simulink model "v2021_10_27_Modello_SITL_AENEA_2020b"  (R2022a)
settings: Solver=ode4  StartTime=0.0  StopTime=10  FixedStep=0.01  RelTol=1e-3
values from neighbouring files (symbols this model uses):
  alphavec_rad = deg2rad(alphavec)    [v2021_10_27_calcoloAerodinamica.m]
  attuatore_Amax = 20*(pi/180)    (= 0.349065850399)    [v2021_10_27_avvioSITL.m]    (also in v2021_10_27_calcoloAerodinamica.m)
  attuatore_Emax = 25*(pi/180)    (= 0.436332312999)    [v2021_10_27_avvioSITL.m]    (also in v2021_10_27_calcoloAerodinamica.m)
  attuatore_Rmax = 25*(pi/180)    (= 0.436332312999)    [v2021_10_27_avvioSITL.m]    (also in v2021_10_27_calcoloAerodinamica.m)
  b = 2.62    [AENEA2.m]    (also in v2021_10_27_calcoloAerodinamica.m)
  betavec_rad = deg2rad(betavec)    [v2021_10_27_calcoloAerodinamica.m]
  c = .32    (= 0.32)    [AENEA2.m]    (also in calcoloPolari.m = dim(2); v2021_10_27_calcoloAerodinamica.m)
  cbar = .32    (= 0.32)    [v2021_10_27_calcoloAerodinamica.m]
  CD0 = 0.024    [v2021_10_27_calcoloAerodinamica.m]
  CldA = KCldA(1)*180/pi    [AENEA2.m]
  CLdE = KCLdE(1)*180/pi    [AENEA2.m]
  CldR = KCldR(1)*180/pi    [AENEA2.m]
  Clp = -0.4318    [v2021_10_27_calcoloAerodinamica.m]
  CLq = 8.13    [v2021_10_27_calcoloAerodinamica.m]
  Clr = 0.1459    [v2021_10_27_calcoloAerodinamica.m]
  CmdE = KCmdE(1)*180/pi    [AENEA2.m]
  Cmq = -23.24    [v2021_10_27_calcoloAerodinamica.m]
  CndA = KCndA(1)*180/pi    [AENEA2.m]
  CndR = KCndR(1)*180/pi    [AENEA2.m]
  Cnp = 0.007507    [v2021_10_27_calcoloAerodinamica.m]
  Cnr = -0.4872    [v2021_10_27_calcoloAerodinamica.m]
  CYp = 0.050728    [v2021_10_27_calcoloAerodinamica.m]
  CYr = 0.358925    [v2021_10_27_calcoloAerodinamica.m]
  deltaAtrim = 0    [v2021_10_27_avvioSITL.m]
  deltaEtrim = 0    [v2021_10_27_avvioSITL.m]
  deltaRtrim = 0    [v2021_10_27_avvioSITL.m]
  deltaTtrim = 0.1    [v2021_10_27_avvioSITL.m]
  Dprop = 2*Rprop    (= 0.5334)    [v2021_10_27_calcoloAerodinamica.m]
  F = [                                     1, 0,            -(dt*vn)/(a + h)^2, dt/(a + h),                     0,   0,  0,  0,  0, 0, 0, 0, 0, 0, 0, 0, 0, 0 ... (first row only)    [jac_F_F1B.m]
  g = [0 0 9.81]'    [v2021_10_27_calcoloAerodinamica.m]
  HINI = -State0.Pos0(3)    [v2021_10_27_avvioSITL.m]
  Jeng = 0    [v2021_10_27_calcoloAerodinamica.m]
  Jprop = mprop*(Dprop^2)/12    (= 0.00422031414)    [v2021_10_27_calcoloAerodinamica.m]
  latitudineINI = 41.854432*pi/180    (= 0.730497644952)    [v2021_10_27_avvioSITL.m]
  longitudineINI = 12.306650*pi/180    (= 0.214791562391)    [v2021_10_27_avvioSITL.m]
  PWM_Aileron = rad2deg(deltaAtrim)*9+1503    [v2021_10_27_avvioSITL.m]
  PWM_Elevator = rad2deg(deltaEtrim)*(447/50)+(3007/2)    [v2021_10_27_avvioSITL.m]
  PWM_Rudder = rad2deg(deltaRtrim)*(447/50)+(3007/2)    [v2021_10_27_avvioSITL.m]
  PWM_Throttle = (deltaTtrim)*800+1100    (= 1180)    [v2021_10_27_avvioSITL.m]
  q = prediction(11)    [jac_F_F1B.m]
  r = dim(1)    [calcoloPolari.m]    (also in jac_F_F1B.m = prediction(12))
  rACtG = rACtP-rGP    [v2021_10_27_calcoloAerodinamica.m]
  rACwG = rACwP-rGP    [v2021_10_27_calcoloAerodinamica.m]
  rAHRSG = rAHRSP-rGP    [v2021_10_27_calcoloAerodinamica.m]
  rho = P/(287.05*T)    (= 1.16123787958)    [AENEA2.m]    (also in modello_appr_long.m = 1.164; v2021_10_27_calcoloAerodinamica.m = 1.2133)
  rLEG = rLEP-rGP    [v2021_10_27_calcoloAerodinamica.m]
  rmglG = rmglP-rGP    [v2021_10_27_calcoloAerodinamica.m]
  rmgrG = rmgrP-rGP    [v2021_10_27_calcoloAerodinamica.m]
  rngG = rngP-rGP    [v2021_10_27_calcoloAerodinamica.m]
  rNPG = rNPP-rGP    [v2021_10_27_calcoloAerodinamica.m]
  rPG = -rGP    [v2021_10_27_calcoloAerodinamica.m]
  Rprop = 0.2667    [v2021_10_27_calcoloAerodinamica.m]
  S = b*c    (= 0.8384)    [AENEA2.m]    (also in v2021_10_27_calcoloAerodinamica.m)
  sensori_FreqCampionamento_pitot = 0.02    [v2021_10_27_avvioSITL.m]
  sensori_RumoreSampleTime = 0.02    [v2021_10_27_avvioSITL.m]
  sensori_varianza = 0.0000    (= 0)    [v2021_10_27_avvioSITL.m]
  tsamp = 0.02    [v2021_10_27_avvioSITL.m]
  V_cruise = input('inserire un valore desiderato per V_cruise [m/s]: ')    [v2021_10_27_trimCalc.m]
  W = m*g    [v2021_10_27_calcoloAerodinamica.m]
  WP_AL = [     0 20 0 0 41.807822 12.589274 3 ... (first row only)    [v2021_10_27_avvioSITL.m]
  WP_db_info = [0 0 0 0 1 3;              0 0 0 0 2 3;              0 0 0 0 3 3;              0 0 0 0 0 0]    [v2021_10_27_avvioSITL.m]
  WP_db_param = [ ... (first row only)    [v2021_10_27_avvioSITL.m]
  Zeng = rPG(3)    [v2021_10_27_calcoloAerodinamica.m]
  Zpista = 0    [v2021_10_27_avvioSITL.m]
undefined symbols (not defined in the file or in its folder): beta_phi, beta_psi, beta_theta, CYdA, CYdR, delay_ahrs, delay_bmp, delay_gps, Earth, h_home, J_vec, matricepolinomi, mean_ax, mean_ay, mean_az, mean_p, mean_q, mean_r, MIL, P_ref, Receive, seed_ahrs, seed_baro, seed_gps, Send, State0, Std_con_lat, Std_con_long, Std_vel, T0_ref, Ta_lat, Ta_long, Ts_ahrs, Ts_bmp, Ts_gps, Var_heading_static, Var_V_hor_static, WGS84, White_ax, White_ay, White_az, White_gm_phi, White_gm_psi, White_gm_theta, White_p, White_pressione, White_r
libraries: simulink_extras x27, aerolibfltsims x5, aerolibwind2 x3, aerolibasang x2, simulink x2, shared6dof x1, slpidlib x1, aerolibatmos2 x1, aerolibanimutils x1
(part 1 of 3)
settings Model: Creator=Giorgio  LastModifiedBy=mvisc
settings SolverCC: AlgebraicLoopSolver=TrustRegion
settings DataIOCC: ReturnWorkspaceOutputs=off
settings DebuggingCC: ParameterPrecisionLossMsg=none  UnconnectedInputMsg=warning  UnconnectedOutputMsg=warning  UnconnectedLineMsg=warning  BusObjectLabelMismatch=none  SFMachineParentedDataDiag=warning  ArithmeticOperatorsInVariantConditions=warning
settings SFSimCC: CustomCodeUndefinedFunction=UseInterfaceOnly
settings RTWCC: DLArmComputeVersion=19.05

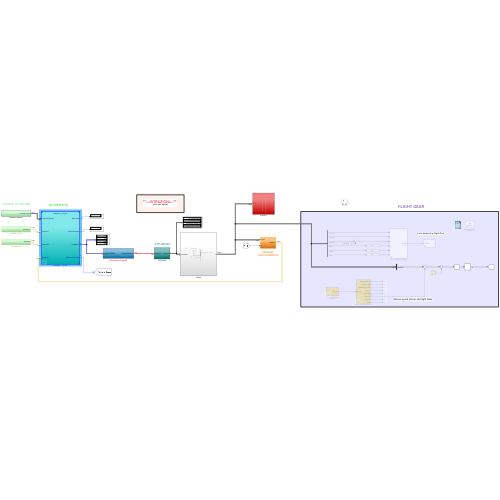
[thumbnail: Simulink's stored preview of the top-level diagram]
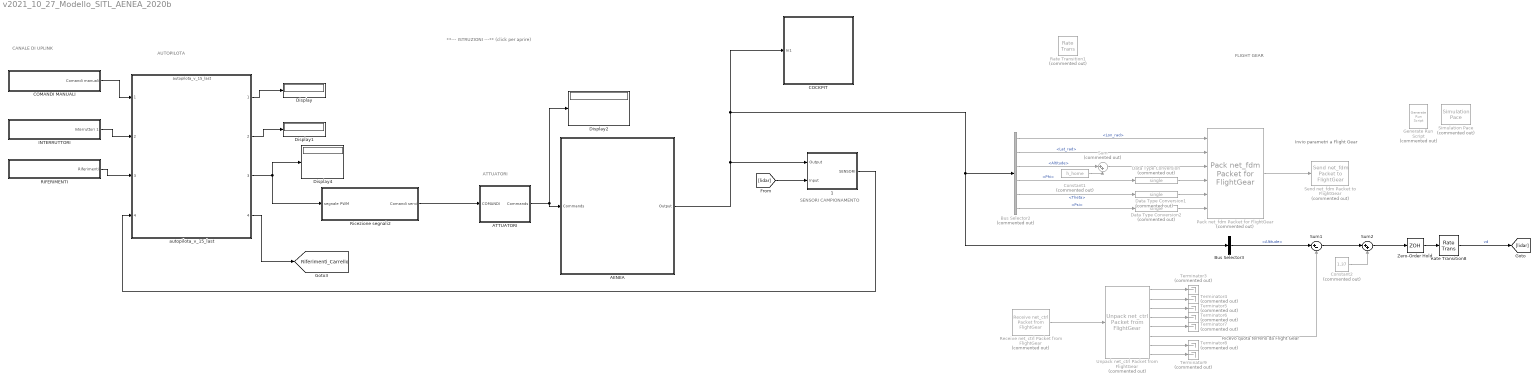
== system v2021_10_27_Modello_SITL_AENEA_2020b ==
  note: AUTOPILOTA
  note: SENSORI
      | CAMPIONAMENTO
  note: ATTUATORI
  note: CANALE DI UPLINK
  note: Ricevo quota terreno da Flight Gear
  note: Invio parametri a Flight Gear
  note: FLIGHT GEAR
  note: **--- ISTRUZIONI ---**
      | (click per aprire)
  " 1" : Subsystem
  "AENEA " : Subsystem
  ATTUATORI : Subsystem
  Bus Selector2 : BusSelector  Commented=on  OutputSignals=Lon_rad,Lat_rad,Altitude,Phi,Theta,Psi
  Bus Selector3 : BusSelector  OutputSignals=Altitude
  COCKPIT : Subsystem
  COMANDI MANUALI : Subsystem
  Constant1 : Constant  Commented=on  Value=h_home
  Constant2 : Constant  Commented=on  Value=1.37
  Data Type Conversion : DataTypeConversion  Commented=on  OutDataTypeStr=single  SaturateOnIntegerOverflow=off  RndMeth=Floor
  Data Type Conversion1 : DataTypeConversion  Commented=on  OutDataTypeStr=single  SaturateOnIntegerOverflow=off  RndMeth=Floor
  Data Type Conversion2 : DataTypeConversion  Commented=on  OutDataTypeStr=single  SaturateOnIntegerOverflow=off  RndMeth=Floor
  Display{,1..2,4} (4 alike) : Display
  Generate Run Script : aerolibfltsims/Generate Run Script  Commented=on  Architecture=Default  dataFlow=Send-Receive  GeometryModelName=c172p  AirportId=LIRF  RunwayId=34L  InitialAltitude=0  InitialHeading=340  OffsetDistance=0  OffsetAzimuth=0  InstallScenery=off  DisableShaders=off  OriginAddress=127.0.0.1  DestinationPort=5502  OriginPort=5505  LocalAddress=127.0.0.1  OutputFileName=runfg_sr.bat  FlightGearBaseDirectory=C:\Program Files\FlightGear 2016.1.2
  "INTERRUTTORI " : Subsystem
  Pack net_fdm Packet for FlightGear : aerolibfltsims/Pack net_fdm Packet for FlightGear  Commented=on  FlightGearVersion=v2016.1  ShowPositionAttitudeInputs=on  ShowVelocityAccelerationInputs=off  ShowControlSurfacePositionInputs=off  ShowEngineFuelInputs=off  ShowLandingGearInputs=off  ShowEnvironmentInputs=off  SampleTime=-1  packetVersion=24
      settings: SourceProductBaseCode=AE
  RIFERIMENTI : Subsystem
  Rate Transition1 : RateTransition  Commented=on  InitialCondition=[PWM_Throttle PWM_Elevator PWM_Aileron PWM_Rudder]
  Rate Transition8 : RateTransition  Deterministic=off  InitialCondition=State0.Pos0(3)  OutPortSampleTime=0.02
  Receive net_ctrl Packet from FlightGear : aerolibfltsims/Receive net_ctrl Packet from FlightGear  Commented=on  FlightGearVersion=v2016.1  ReceiveAddress=127.0.0.1  ReceivePort=5505  ReceiveWidth=744  varLen=off  SampleTime=-1  packetFlag=off
      settings: AttributesFormatString=Version Selected:\n%<FlightGearVersion>  SourceProductBaseCode=AE
  Ricezione segnali2 : Subsystem
  Send net_fdm Packet to FlightGear : aerolibfltsims/Send net_fdm Packet to FlightGear  Commented=on  DestinationIpAddress=127.0.0.1  DestinationPort=5502  LocalIpPort=-1  varLen=off  SampleTime=-1
      settings: SourceProductBaseCode=AE
  Simulation Pace : aerolibanimutils/Simulation Pace  Commented=on  SimulationPace=1  SleepMode=MATLAB Thread  OutputPaceError=off  SampleTime=tsamp
  Sum : Sum  Commented=on  Inputs=|++
  Sum1 : Sum  Inputs=|+-
  Sum2 : Sum  Inputs=|++
  Terminator{3..9} (7 alike) : Terminator  Commented=on
  Unpack net_ctrl Packet from FlightGear : aerolibfltsims/Unpack net_ctrl Packet from FlightGear  Commented=on  FlightGearVersion=v2016.1  ShowControlSurfacePositionOutputs=off  ShowEngineFuelOutputs=off  ShowLandingGearOutputs=off  ShowAvionicOutputs=off  ShowEnvironmentOutputs=on  SampleTime=-1  packetVersion=27
      settings: AttributesFormatString=Version Selected: %<FlightGearVersion>  SourceProductBaseCode=AE
  Zero-Order Hold : ZeroOrderHold  SampleTime=0.02
  autopilota_v_15_last : ModelReference  ModelNameDialog=autopilota_v_15_last.slx  SimulationMode=Normal  ModelReferenceVersion=8.0
  tag scope: Riferimenti_Carrello=global
  wires:
  autopilota_v_15_last/1 -> Display/1
  "INTERRUTTORI "/1(Interruttori 1) -> autopilota_v_15_last/2
  COMANDI MANUALI/1(Comandi manuali) -> autopilota_v_15_last/1
  autopilota_v_15_last/2 -> Display1/1
  RIFERIMENTI/1(Riferimenti) -> autopilota_v_15_last/3
  Constant2/1 -> Sum2/2
  Bus Selector2/6 -> Data Type Conversion2/1  "<Psi>"
  Bus Selector2/3 -> Sum/1  "<Altitude>"
  Sum1/1 -> Sum2/1
  Unpack net_ctrl Packet from FlightGear/6 -> Sum1/2
  Unpack net_ctrl Packet from FlightGear/2 -> Terminator4/1
  Unpack net_ctrl Packet from FlightGear/7 -> Terminator8/1
  Rate Transition8/1 -> [lidar]  "vd"
  Receive net_ctrl Packet from FlightGear/1 -> Unpack net_ctrl Packet from FlightGear/1
  Sum2/1 -> Zero-Order Hold/1
  Unpack net_ctrl Packet from FlightGear/8 -> Terminator9/1
  Bus Selector2/2 -> Pack net_fdm Packet for FlightGear/2  "<Lat_rad>"
  Constant1/1 -> Sum/2
  Data Type Conversion2/1 -> Pack net_fdm Packet for FlightGear/6
  Bus Selector3/1 -> Sum1/1  "<Altitude>"
  Unpack net_ctrl Packet from FlightGear/3 -> Terminator5/1
  Pack net_fdm Packet for FlightGear/1 -> Send net_fdm Packet to FlightGear/1
  Zero-Order Hold/1 -> Rate Transition8/1
  Data Type Conversion/1 -> Pack net_fdm Packet for FlightGear/4
  Sum/1 -> Pack net_fdm Packet for FlightGear/3
  Bus Selector2/4 -> Data Type Conversion/1  "<Phi>"
  Bus Selector2/5 -> Data Type Conversion1/1  "<Theta>"
  Unpack net_ctrl Packet from FlightGear/1 -> Terminator3/1
  Data Type Conversion1/1 -> Pack net_fdm Packet for FlightGear/5
  Bus Selector2/1 -> Pack net_fdm Packet for FlightGear/1  "<Lon_rad>"
  Unpack net_ctrl Packet from FlightGear/4 -> Terminator6/1
  Unpack net_ctrl Packet from FlightGear/5 -> Terminator7/1
  [lidar] -> " 1"/2(Input)
  "AENEA "/1(Output) -> " 1"/1(Output), Bus Selector3/1, Bus Selector2/1, COCKPIT/1(In1)
  ATTUATORI/1(Commands) -> "AENEA "/1(Commands), Display2/1
  autopilota_v_15_last/3 -> Display4/1, Ricezione segnali2/1(segnale PWM)
  Ricezione segnali2/1(Comandi servi) -> ATTUATORI/1("COMANDI ")
  " 1"/1(SENSORI) -> autopilota_v_15_last/4
  autopilota_v_15_last/4 -> [Riferimenti_Carrello]

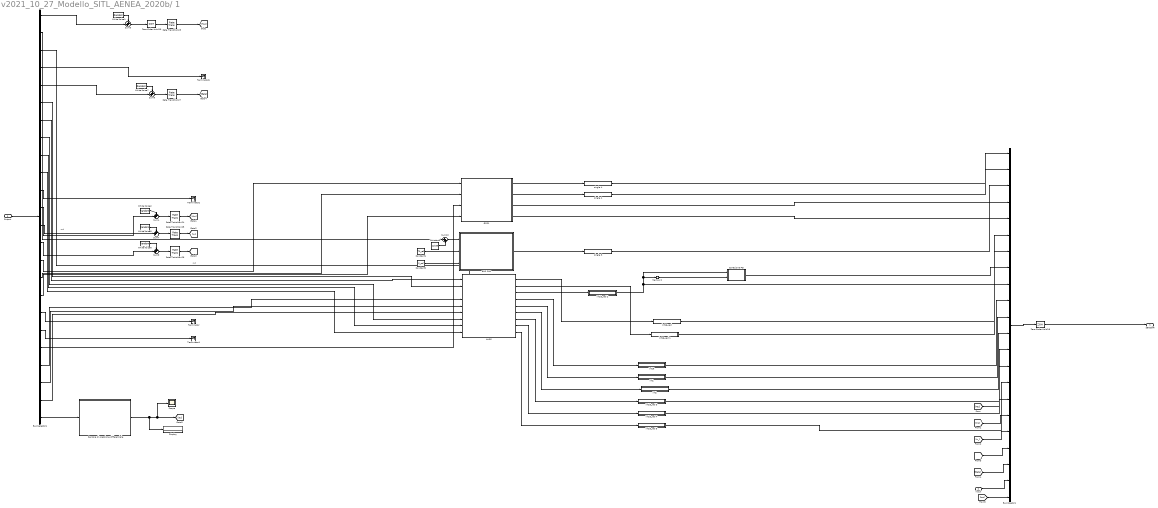
== system v2021_10_27_Modello_SITL_AENEA_2020b/ 1 ==
  note: rad
  note: rad
  Output : Inport
  Input : Inport  Port=2
  AHRS : Subsystem
  BMP 280 : Subsystem
  Bus Creator1 : BusCreator  Inputs=22  OutDataTypeStr=Bus: slBus8_sensori2
  Bus Selector1 : BusSelector  OutputSignals=V,Altitude,Psi,α,β,Theta,Phi,p,q,r,Zepunto,rho,w,Omega,Lat_rad,Lon_rad,heading,Xepunto,Yepunto,GS,upunto,vpunto,wpunto,deltaP
  Constant1 : Constant  Value=T0_ref
  Constant2 : Constant  Value=P_ref
  Constant3 : Constant  Value=Zpista
  Correzione PSI : MATLAB Function  TreatAsAtomicUnit=on
  Display : Display
  GPS1 : Subsystem
  Memory2 : Memory
  Rate Transition23 : RateTransition  OutPortSampleTime=0.02
  Rate Transition{24..27} (4 alike) : RateTransition  OutPortSampleTimeOpt=Inherit
  Scope : Scope
  Sensore di pressione differenziale : Subsystem
  Sum10 : Sum  Inputs=|++
  Sum{3..4,7..9} (5 alike) : Sum  Inputs=++|
  Terminator{,1..2,6} (4 alike) : Terminator
  White Noise1 : RandomNumber  DisableCoverage=on  Variance=1e-1  Seed=[23341]  SampleTime=sensori_RumoreSampleTime
  White Noise{2,5..7} (4 alike) : RandomNumber  DisableCoverage=on  Variance=sensori_varianza  Seed=[23341]  SampleTime=sensori_RumoreSampleTime
  Zero-Order Hold18 : ZeroOrderHold  SampleTime=0.02
  Zero-Order Hold19 : ZeroOrderHold  SampleTime=sensori_FreqCampionamento_pitot
  int1 : Subsystem
  int16 : Subsystem
  "int16_rad " : Subsystem
  int16_rad 1 : Subsystem
  int16_rad 2 : Subsystem
  int16_rad 3 : Subsystem
  int16_rad 4 : Subsystem
  int16_rad 5 : Subsystem
  int2 : Subsystem
  single 1 : Subsystem
  single 3 : Subsystem
  single 4 : Subsystem
  SENSORI : Outport  OutDataTypeStr=double  VectorParamsAs1DForOutWhenUnconnected=off
  wires:
  GPS1/3(V_n) -> Bus Creator1/4  "vn"
  Bus Selector1/19 -> Terminator1/1  "<Yepunto>"
  Bus Selector1/6 -> AHRS/2(theta)  "<Theta>"
  Bus Selector1/4 -> Terminator6/1  "<α>"
  Bus Selector1/23 -> AHRS/6(az)  "<wpunto>"
  Bus Selector1/18 -> Terminator/1  "<Xepunto>"
  Bus Selector1/2 -> Sum10/1  "<Altitude>"
  Bus Selector1/16 -> GPS1/2(Long)  "<Lon_rad>"
  Bus Selector1/17 -> GPS1/4(head)  "<heading>"
  Bus Selector1/7 -> AHRS/1(phi)  "<Phi>"
  Bus Selector1/22 -> AHRS/5(ay)  "<vpunto>"
  Bus Selector1/10 -> AHRS/9(r)  "<r>"
  GPS1/1(Lat_out) -> single 4/1(<u>)  "Lat"
  Rate Transition27/1 -> [Beta]  "Beta"
  "int16_rad "/1(Out1) -> Bus Creator1/6  "phi"
  Bus Selector1/5 -> Sum9/2  "<β>"
  White Noise2/1 -> Sum4/1
  White Noise5/1 -> Sum7/1
  AHRS/7(p_out) -> int16_rad 3/1(In1)  "p"
  Sum4/1 -> Rate Transition24/1  "rho"
  int16/1(Out1) -> Bus Creator1/10  "ax"
  Bus Selector1/14 -> Sum8/2  "<Omega>"
  BMP 280/1(quota_out) -> single 3/1(<u>)  "Alt"
  AHRS/4(ax_out) -> int16/1(In1)  "ax"
  Rate Transition25/1 -> [w_]  "w"
  int16_rad 5/1(Out1) -> Bus Creator1/15  "r"
  AHRS/6(az_out) -> int2/1(In1)  "az"
  GPS1/4(V_e) -> Bus Creator1/5  "ve"
  Bus Selector1/12 -> Sum4/2  "<rho>"
  Constant1/1 -> BMP 280/2(T0_ref)
  Bus Selector1/8 -> AHRS/7(p)  "<p>"
  Sum7/1 -> Rate Transition25/1  "w"
  Output/1 -> Bus Selector1/1
  Sum3/1 -> Zero-Order Hold19/1  "Tas"
  Bus Selector1/11 -> Terminator2/1  "<Zepunto>"
  AHRS/1(phi_out) -> "int16_rad "/1(In1)  "phi"
  Bus Selector1/9 -> AHRS/8(q)  "<q>"
  Bus Selector1/21 -> AHRS/4(ax)  "<upunto>"
  Bus Selector1/3 -> AHRS/3(psi)  "<Psi>"
  int16_rad 3/1(Out1) -> Bus Creator1/13  "p"
  Rate Transition23/1 -> [Tas]  "Tas"
  AHRS/9(r_out) -> int16_rad 5/1(In1)  "r"
  int16_rad 4/1(Out1) -> Bus Creator1/14  "q"
  White Noise1/1 -> Sum3/1
  int2/1(Out1) -> Bus Creator1/12  "az"
  Bus Selector1/20 -> GPS1/3(vel)  "<GS>"
  Memory2/1 -> Correzione PSI/2(psi_k)
  White Noise6/1 -> Sum8/1
  Zero-Order Hold19/1 -> Rate Transition23/1  "Tas"
  AHRS/2(theta_out) -> int16_rad 1/1(In1)  "theta"
  AHRS/8(q_out) -> int16_rad 4/1(In1)  "q"
  int1/1(Out1) -> Bus Creator1/11  "ay"
  single 3/1(Out1) -> Bus Creator1/3  "Quota"
  GPS1/2("Long_out ") -> single 1/1(<u>)  "Long"
  AHRS/5(ay_out) -> int1/1(In1)  "ay"
  single 1/1(Out1) -> Bus Creator1/2  "Long"
  Rate Transition24/1 -> [rho]  "rho"
  White Noise7/1 -> Sum9/1
  Sum10/1 -> BMP 280/1(quota)
  Bus Selector1/15 -> GPS1/1(Lat)  "<Lat_rad>"
  Constant2/1 -> BMP 280/3(P_ref)
  Rate Transition26/1 -> [omega]  "omega"
  Bus Selector1/1 -> Sum3/2  "<V>"
  Bus Selector1/13 -> Sum7/2  "<w>"
  Sum8/1 -> Rate Transition26/1  "omega"
  int16_rad 1/1(Out1) -> Bus Creator1/7  "theta"
  Sum9/1 -> Rate Transition27/1  "Beta"
  AHRS/3(psi_out) -> int16_rad 2/1(In1)  "psi"
  Zero-Order Hold18/1 -> SENSORI/1
  int16_rad 2/1(Out1) -> Memory2/1, Correzione PSI/1(psi), Bus Creator1/9  "psi"
  Constant3/1 -> Sum10/2
  single 4/1(Out1) -> Bus Creator1/1  "Lat"
  [Tas] -> Bus Creator1/16
  [rho] -> Bus Creator1/17
  [w_] -> Bus Creator1/18
  [omega] -> Bus Creator1/19
  [Beta] -> Bus Creator1/20
  Input/1 -> Bus Creator1/21
  Bus Creator1/1 -> Zero-Order Hold18/1
  Correzione PSI/1(y) -> Bus Creator1/8  "psi_non_corretta"
  Sensore di pressione differenziale/1(Out1) -> Display/1, [Ias], Scope/1  "Ias"
  Bus Selector1/24 -> Sensore di pressione differenziale/1(In1)  "<deltaP>"
  [Ias] -> Bus Creator1/22

== system v2021_10_27_Modello_SITL_AENEA_2020b/AENEA  ==
  Commands : Inport  OutDataTypeStr=double
  AENEA II_SITL1 : Subsystem
  Blocco_Costanti1 : Subsystem
  Bus Creator : BusCreator  Inputs=4
  Bus Creator1 : BusCreator  Inputs=4
  Bus Selector : BusSelector  OutputSignals=deltaE,deltaA,deltaR,Manetta
  Bus Selector1 : BusSelector  OutputSignals=xyz.h
  Bus Selector2 : BusSelector  OutputSignals=Vbpolare.V
  Constant : Constant  Value=[0,0,0]
  Constant1 : Constant  Value=rho
  Constant2 : Constant  Value=1/2
  Gain : Gain  Gain=-1
  ISA Atmosphere Model : aerolibatmos2/ISA Atmosphere Model  custom=off  g=9.80665  gamma=1.4  R=287.0531  L=0.0065  h_trop=11000  h_strat=20000  rho0=1.225  P0=101325  T0=288.15  h0=0
  Product : Product  Inputs=3
  Square : Math  Operator=square
  Terminator : Terminator
  Terminator1 : Terminator
  Terminator2 : Terminator
  toSensors : Subsystem
  Output : Outport  VectorParamsAs1DForOutWhenUnconnected=off
  wires:
  Bus Selector/2 -> Bus Creator/2  "<deltaA>"
  Blocco_Costanti1/1(Vect_Costanti) -> AENEA II_SITL1/2(Vect_Costanti), Bus Creator1/4  "Costanti"
  Bus Creator/1 -> AENEA II_SITL1/1(Vect_Comandi)
  Gain/1 -> ISA Atmosphere Model/1
  Bus Selector/4 -> Bus Creator/4  "<Manetta>"
  Bus Selector/1 -> Bus Creator/1  "<deltaE>"
  Bus Selector/3 -> Bus Creator/3  "<deltaR>"
  ISA Atmosphere Model/2 -> Terminator1/1
  ISA Atmosphere Model/1 -> Terminator2/1
  Constant/1 -> AENEA II_SITL1/4(Constant Wind)  "Constant Wind"
  Commands/1 -> Bus Selector/1
  Bus Selector1/1 -> Gain/1  "<h>"
  Bus Creator1/1 -> toSensors/1("[X,Y,Xpunto,Costanti]")
  AENEA II_SITL1/3(Xpunto) -> Bus Creator1/3  "Xpunto"
  AENEA II_SITL1/1(Xstato) -> Bus Creator1/1, Bus Selector1/1  "X"
  ISA Atmosphere Model/3 -> Terminator/1
  toSensors/1(Out_to_campionamento) -> Output/1
  Constant1/1 -> AENEA II_SITL1/3(ρ)
  Square/1 -> Product/3
  AENEA II_SITL1/2(Y) -> Bus Creator1/2, Bus Selector2/1  "Y"
  Constant2/1 -> Product/2
  Product/1 -> toSensors/3(deltaP)  "deltaP"
  ISA Atmosphere Model/4 -> Product/1, toSensors/2(rho)
  Bus Selector2/1 -> Square/1  "<V>"

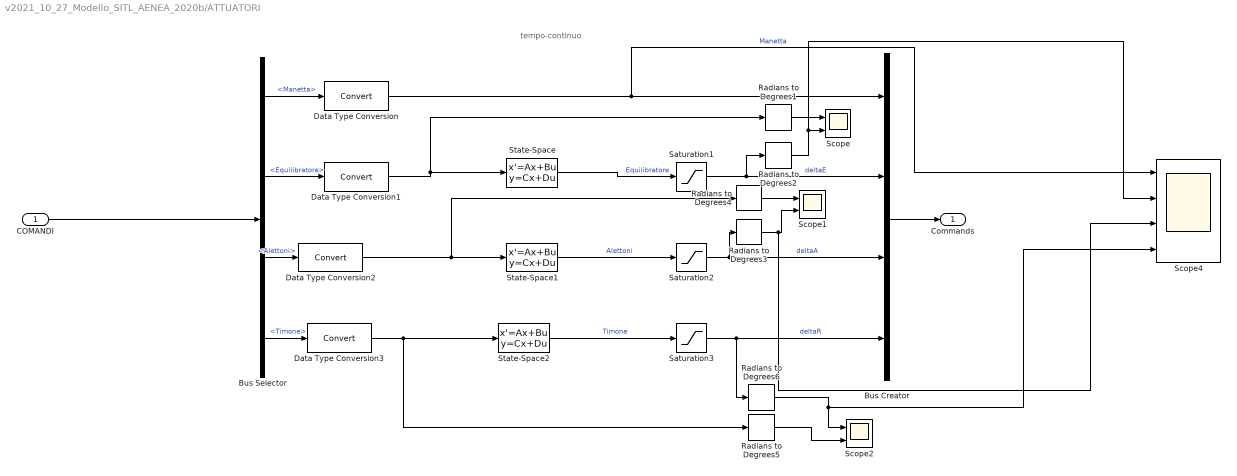
== system v2021_10_27_Modello_SITL_AENEA_2020b/ATTUATORI ==
  note: tempo-continuo
  "COMANDI " : Inport
  Bus Creator : BusCreator  Inputs=4
  Bus Selector : BusSelector  OutputSignals=Manetta,Equilibratore,Alettoni,Timone
  Data Type Conversion{,1..3} (4 alike) : DataTypeConversion  SaturateOnIntegerOverflow=off  RndMeth=Floor
  Radians to Degrees{1..6} (6 alike) : simulink_extras/Transformations/Radians to Degrees
  Saturation1 : Saturate  UpperLimit=attuatore_Emax+0.1  LowerLimit=-attuatore_Emax
  Saturation2 : Saturate  UpperLimit=attuatore_Amax+0.1  LowerLimit=-attuatore_Amax
  Saturation3 : Saturate  UpperLimit=attuatore_Rmax+0.1  LowerLimit=-attuatore_Rmax
  Scope : Scope  NumInputPorts=2
  Scope1 : Scope  NumInputPorts=2
  Scope2 : Scope  NumInputPorts=2
  Scope4 : Scope  NumInputPorts=4
  State-Space : StateSpace  A=-12.54  C=12.54  D=0  InitialCondition=State0.Ele0
  State-Space1 : StateSpace  A=-12.54  C=12.54  D=0  InitialCondition=State0.Ail0
  State-Space2 : StateSpace  A=-12.54  C=12.54  D=0  InitialCondition=State0.Rud0
  Commands : Outport  VectorParamsAs1DForOutWhenUnconnected=off
  wires:
  "COMANDI "/1 -> Bus Selector/1
  Radians to Degrees3/1 -> Scope4/3, Scope1/2
  Bus Selector/2 -> Data Type Conversion1/1  "<Equilibratore>"
  State-Space/1 -> Saturation1/1  "Equilibratore"
  Radians to Degrees1/1 -> Scope/1
  Radians to Degrees4/1 -> Scope1/1
  Saturation2/1 -> Radians to Degrees3/1, Bus Creator/3  "deltaA"
  Saturation1/1 -> Bus Creator/2, Radians to Degrees2/1  "deltaE"
  Bus Selector/1 -> Data Type Conversion/1  "<Manetta>"
  Saturation3/1 -> Radians to Degrees6/1, Bus Creator/4  "deltaR"
  Bus Creator/1 -> Commands/1
  Radians to Degrees6/1 -> Scope4/4, Scope2/1
  Bus Selector/3 -> Data Type Conversion2/1  "<Alettoni>"
  Radians to Degrees2/1 -> Scope4/2, Scope/2
  Bus Selector/4 -> Data Type Conversion3/1  "<Timone>"
  State-Space2/1 -> Saturation3/1  "Timone"
  State-Space1/1 -> Saturation2/1  "Alettoni"
  Radians to Degrees5/1 -> Scope2/2
  Data Type Conversion/1 -> Scope4/1, Bus Creator/1  "Manetta"
  Data Type Conversion1/1 -> State-Space/1, Radians to Degrees1/1
  Data Type Conversion2/1 -> State-Space1/1, Radians to Degrees4/1
  Data Type Conversion3/1 -> State-Space2/1, Radians to Degrees5/1

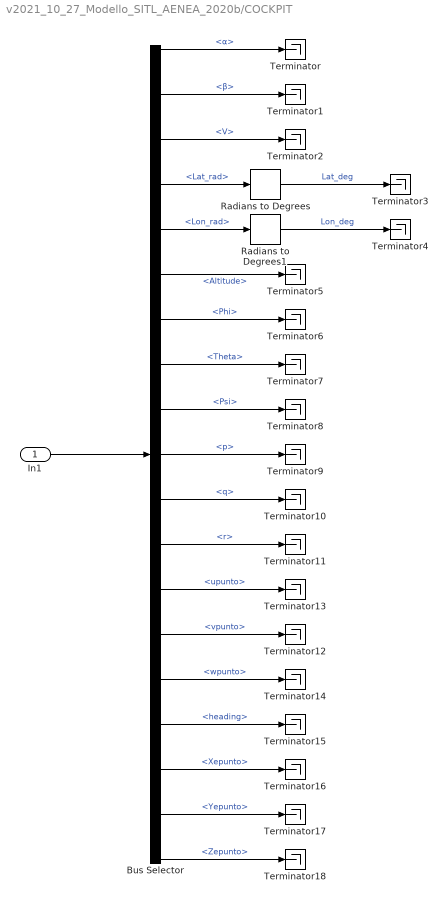
== system v2021_10_27_Modello_SITL_AENEA_2020b/COCKPIT ==
  In1 : Inport
  Bus Selector : BusSelector  OutputSignals=α,β,V,Lat_rad,Lon_rad,Altitude,Phi,Theta,Psi,p,q,r,upunto,vpunto,wpunto,heading,Xepunto,Yepunto,Zepunto
  Radians to Degrees : simulink_extras/Transformations/Radians to Degrees
  Radians to Degrees1 : simulink_extras/Transformations/Radians to Degrees
  Terminator{,1..18} (19 alike) : Terminator
  wires:
  In1/1 -> Bus Selector/1
  Bus Selector/1 -> Terminator/1  "<α>"
  Bus Selector/2 -> Terminator1/1  "<β>"
  Bus Selector/3 -> Terminator2/1  "<V>"
  Bus Selector/4 -> Radians to Degrees/1  "<Lat_rad>"
  Bus Selector/5 -> Radians to Degrees1/1  "<Lon_rad>"
  Bus Selector/6 -> Terminator5/1  "<Altitude>"
  Bus Selector/7 -> Terminator6/1  "<Phi>"
  Bus Selector/8 -> Terminator7/1  "<Theta>"
  Bus Selector/9 -> Terminator8/1  "<Psi>"
  Bus Selector/10 -> Terminator9/1  "<p>"
  Bus Selector/11 -> Terminator10/1  "<q>"
  Bus Selector/12 -> Terminator11/1  "<r>"
  Bus Selector/13 -> Terminator13/1  "<upunto>"
  Bus Selector/14 -> Terminator12/1  "<vpunto>"
  Bus Selector/15 -> Terminator14/1  "<wpunto>"
  Bus Selector/16 -> Terminator15/1  "<heading>"
  Bus Selector/17 -> Terminator16/1  "<Xepunto>"
  Bus Selector/18 -> Terminator17/1  "<Yepunto>"
  Bus Selector/19 -> Terminator18/1  "<Zepunto>"
  Radians to Degrees1/1 -> Terminator4/1  "Lon_deg"
  Radians to Degrees/1 -> Terminator3/1  "Lat_deg"

== system v2021_10_27_Modello_SITL_AENEA_2020b/COMANDI MANUALI ==
  A : Constant  Value=deltaAtrim  SampleTime=0.02
  Bus Creator3 : BusCreator  Inputs=5  OutDataTypeStr=Bus: slBus4_manuali
  Constant : Constant
  Constant1 : Constant  Value=0
  Constant2 : Constant  Commented=on  Value=0
  E : Constant  Value=deltaEtrim  SampleTime=0.02
  R : Constant  Value=deltaRtrim  SampleTime=0.02
  Switch : Switch  Criteria=u2 > Threshold  Threshold=1500  SaturateOnIntegerOverflow=off  InputSameDT=off
  T : Constant  Value=deltaTtrim  SampleTime=0.02
  cg_home4 : Constant  Value=0
  Comandi manuali : Outport  VectorParamsAs1DForOutWhenUnconnected=off
  wires:
  A/1 -> Bus Creator3/2  "Manual_Aileron"
  E/1 -> Bus Creator3/1  "Manual_Elevator"
  T/1 -> Bus Creator3/4  "Manual_Throttle"
  cg_home4/1 -> Switch/2
  Constant/1 -> Switch/1
  Constant1/1 -> Switch/3
  Switch/1 -> Bus Creator3/5  "Go_Home"
  Bus Creator3/1 -> Comandi manuali/1  "Comandi manuali"
  R/1 -> Bus Creator3/3  "Manual_Rudder"

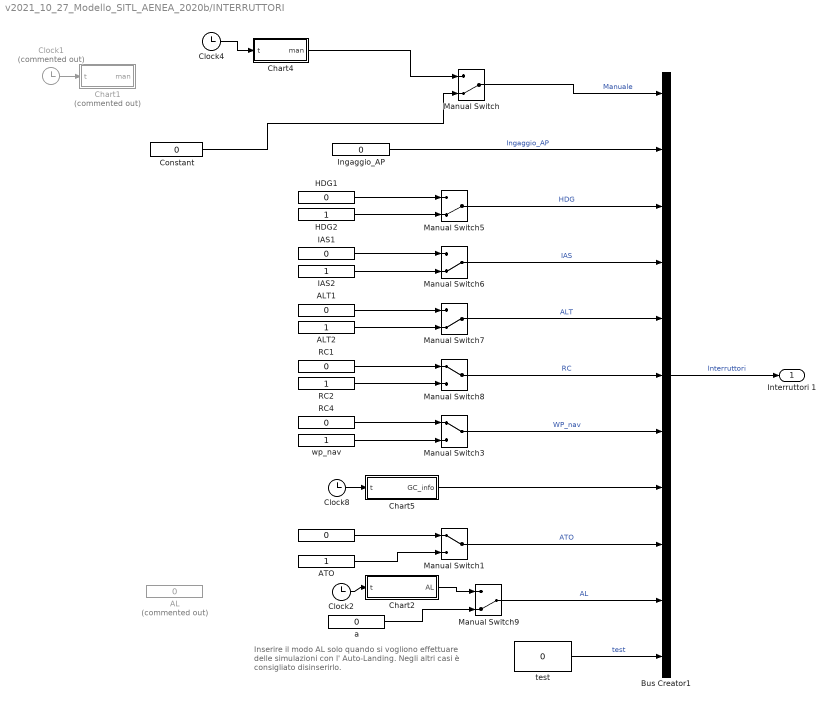
== system v2021_10_27_Modello_SITL_AENEA_2020b/INTERRUTTORI  ==
  note: Inserire il modo AL solo quando si vogliono effettuare
      | delle simulazioni con l' Auto-Landing. Negli altri casi è
      | consigliato disinserirlo.
  " " : Constant  Value=0
  AL : Constant  Commented=on  Value=0
  ALT1 : Constant  Value=0
  ALT2 : Constant
  ATO : Constant
  Bus Creator1 : BusCreator  Inputs=11
  Chart1 : Stateflow chart  Commented=on  TreatAsAtomicUnit=on
  Chart2 : Stateflow chart  TreatAsAtomicUnit=on
  "Chart4 " : Stateflow chart  TreatAsAtomicUnit=on
  Chart5 : Stateflow chart  TreatAsAtomicUnit=on
  Clock1 : Clock  Commented=on
  Clock2 : Clock
  Clock4 : Clock
  Clock8 : Clock
  Constant : Constant  Value=0
  HDG1 : Constant  Value=0
  HDG2 : Constant
  IAS1 : Constant  Value=0
  IAS2 : Constant
  Ingaggio_AP : Constant  Value=0
  Manual Switch{,5..7,9} (5 alike) : ManualSwitch  CurrentSetting=0
  Manual Switch1 : ManualSwitch
  Manual Switch3 : ManualSwitch
  Manual Switch8 : ManualSwitch
  RC1 : Constant  Value=0
  RC2 : Constant
  RC4 : Constant  Value=0
  a : Constant  Value=0
  test : Constant  Value=0
  wp_nav : Constant
  Interruttori 1 : Outport  VectorParamsAs1DForOutWhenUnconnected=off
  wires:
  Ingaggio_AP/1 -> Bus Creator1/2  "Ingaggio_AP"
  Bus Creator1/1 -> Interruttori 1/1  "Interruttori"
  Manual Switch7/1 -> Bus Creator1/5  "ALT"
  Manual Switch6/1 -> Bus Creator1/4  "IAS"
  Manual Switch5/1 -> Bus Creator1/3  "HDG"
  Clock8/1 -> Chart5/1(t)
  Chart5/1(GC_info) -> Bus Creator1/8
  Manual Switch3/1 -> Bus Creator1/7  "WP_nav"
  Manual Switch8/1 -> Bus Creator1/6  "RC"
  test/1 -> Bus Creator1/11  "test"
  Manual Switch1/1 -> Bus Creator1/9  "ATO"
  IAS1/1 -> Manual Switch6/1
  IAS2/1 -> Manual Switch6/2
  HDG2/1 -> Manual Switch5/2
  HDG1/1 -> Manual Switch5/1
  RC4/1 -> Manual Switch3/1
  wp_nav/1 -> Manual Switch3/2
  RC2/1 -> Manual Switch8/2
  RC1/1 -> Manual Switch8/1
  ALT1/1 -> Manual Switch7/1
  Manual Switch9/1 -> Bus Creator1/10  "AL"
  ALT2/1 -> Manual Switch7/2
  Clock1/1 -> Chart1/1(t)
  Clock4/1 -> "Chart4 "/1(t)
  Manual Switch/1 -> Bus Creator1/1  "Manuale"
  "Chart4 "/1(man) -> Manual Switch/1
  ATO/1 -> Manual Switch1/2
  " "/1 -> Manual Switch1/1
  a/1 -> Manual Switch9/2
  Clock2/1 -> Chart2/1(t)
  Chart2/1(AL) -> Manual Switch9/1
  Constant/1 -> Manual Switch/2

== system v2021_10_27_Modello_SITL_AENEA_2020b/RIFERIMENTI ==
  Bus Creator1 : BusCreator  Inputs=7
  Chart1 : Stateflow chart  TreatAsAtomicUnit=on
  Chart2 : Stateflow chart  TreatAsAtomicUnit=on
  Chart3 : Stateflow chart  Commented=on  TreatAsAtomicUnit=on
  Clock1 : Clock
  Clock2 : Clock
  Clock3 : Clock  Commented=on
  Manual Switch : ManualSwitch  CurrentSetting=0
  Manual Switch1 : ManualSwitch  CurrentSetting=0
  Manual Switch2 : ManualSwitch  CurrentSetting=0
  QUOTA (m) : Constant  Value=100
  RC (ft/min) : Constant  Value=0
  ROTTA  ( ° ) : Constant  Value=0
  VELOCITA'  (m/s) : Constant  Value=25
  WP_AL : Constant  Value=WP_AL
  WP_db_info : Constant  Value=WP_db_info
  WP_db_param : Constant  Value=WP_db_param
  ft/min2m/s : Gain  Gain=0.00508
  Riferimenti : Outport  VectorParamsAs1DForOutWhenUnconnected=off
  wires:
  VELOCITA'  (m/s)/1 -> Manual Switch2/2  "VELOCITA"
  Bus Creator1/1 -> Riferimenti/1  "Riferimenti"
  RC (ft/min)/1 -> ft/min2m/s/1  "RC"
  WP_db_info/1 -> Bus Creator1/5  "WP_db_info"
  WP_db_param/1 -> Bus Creator1/6  "WP_db_param"
  Clock2/1 -> Chart2/1(t)
  Chart2/1(ROTTA) -> Manual Switch/1  "ROTTA"
  Clock1/1 -> Chart1/1(t)
  Chart1/1(QUOTA) -> Manual Switch1/1
  ROTTA  ( ° )/1 -> Manual Switch/2  "ROTTA"
  Manual Switch/1 -> Bus Creator1/1  "ROTTA"
  QUOTA (m)/1 -> Manual Switch1/2  "QUOTA"
  Manual Switch1/1 -> Bus Creator1/3  "QUOTA"
  WP_AL/1 -> Bus Creator1/7  "WP_AL"
  Chart3/1(ROTTA) -> Manual Switch2/1  "VEL"
  Clock3/1 -> Chart3/1(t)
  Manual Switch2/1 -> Bus Creator1/2  "VELOCITA"
  ft/min2m/s/1 -> Bus Creator1/4

== system v2021_10_27_Modello_SITL_AENEA_2020b/Ricezione segnali2 ==
  segnale PWM : Inport
  Bus Creator3 : BusCreator  Inputs=4
  Delay : Delay  InitialCondition=PWM_Throttle
  Delay1 : Delay  InitialCondition=PWM_Elevator
  Delay2 : Delay  InitialCondition=PWM_Aileron
  Delay3 : Delay  InitialCondition=PWM_Rudder
  Demux : Demux
  Display : Display
  Subsystem1 : Subsystem  TreatAsAtomicUnit=on  SystemSampleTime=0.01
  Comandi servi : Outport  VectorParamsAs1DForOutWhenUnconnected=off
  wires:
  segnale PWM/1 -> Demux/1
  Bus Creator3/1 -> Comandi servi/1  "Comandi manuali"
  Demux/1 -> Delay/1
  Demux/2 -> Delay1/1
  Demux/3 -> Delay2/1
  Demux/4 -> Delay3/1
  Subsystem1/1(Out1) -> Bus Creator3/1
  Subsystem1/3(Out3) -> Bus Creator3/3
  Subsystem1/4(Out4) -> Bus Creator3/4
  Delay/1 -> Subsystem1/1(In1)
  Delay1/1 -> Subsystem1/2(In2)
  Delay2/1 -> Subsystem1/3(In3)
  Delay3/1 -> Subsystem1/4(In4)
  Subsystem1/2(Out2) -> Display/1, Bus Creator3/2

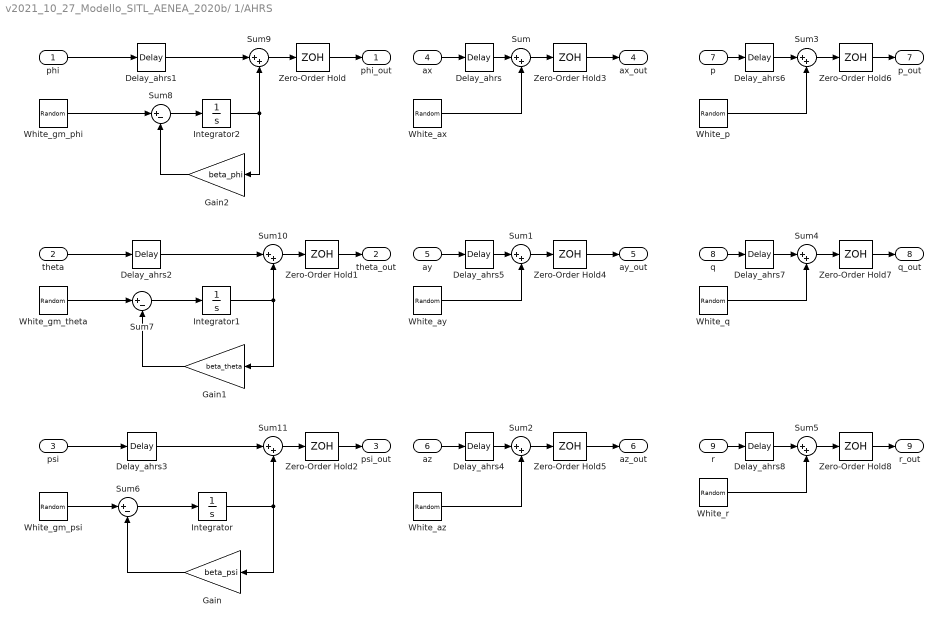
== system v2021_10_27_Modello_SITL_AENEA_2020b/ 1/AHRS ==
  phi : Inport
  theta : Inport  Port=2
  psi : Inport  Port=3
  ax : Inport  Port=4
  ay : Inport  Port=5
  az : Inport  Port=6
  p : Inport  Port=7
  q : Inport  Port=8
  r : Inport  Port=9
  Delay_ahrs{,1..8} (9 alike) : TransportDelay  DelayTime=delay_ahrs
  Gain : Gain  Gain=beta_psi  SaturateOnIntegerOverflow=on  OutDataTypeStr=Inherit: Same as input  ParamDataTypeStr=Inherit: Same as input
  Gain1 : Gain  Gain=beta_theta  SaturateOnIntegerOverflow=on  OutDataTypeStr=Inherit: Same as input  ParamDataTypeStr=Inherit: Same as input
  Gain2 : Gain  Gain=beta_phi  SaturateOnIntegerOverflow=on  OutDataTypeStr=Inherit: Same as input  ParamDataTypeStr=Inherit: Same as input
  Integrator : Integrator
  Integrator1 : Integrator
  Integrator2 : Integrator
  Sum{,1..5} (6 alike) : Sum  Inputs=|++
  Sum10 : Sum  Inputs=|++  InputSameDT=on  SaturateOnIntegerOverflow=on  OutDataTypeStr=Inherit: Same as first input
  Sum11 : Sum  Inputs=|++  InputSameDT=on  SaturateOnIntegerOverflow=on  OutDataTypeStr=Inherit: Same as first input
  Sum6 : Sum  Inputs=|+-  InputSameDT=on  SaturateOnIntegerOverflow=on  OutDataTypeStr=Inherit: Same as first input
  Sum7 : Sum  Inputs=|+-  InputSameDT=on  SaturateOnIntegerOverflow=on  OutDataTypeStr=Inherit: Same as first input
  Sum8 : Sum  Inputs=|+-  InputSameDT=on  SaturateOnIntegerOverflow=on  OutDataTypeStr=Inherit: Same as first input
  Sum9 : Sum  Inputs=|++  InputSameDT=on  SaturateOnIntegerOverflow=on  OutDataTypeStr=Inherit: Same as first input
  White_ax : RandomNumber  Mean=mean_ax  Variance=White_ax  Seed=seed_ahrs  SampleTime=Ts_ahrs
  White_ay : RandomNumber  Mean=mean_ay  Variance=White_ay  Seed=seed_ahrs  SampleTime=Ts_ahrs
  White_az : RandomNumber  Mean=mean_az  Variance=White_az  Seed=seed_ahrs  SampleTime=Ts_ahrs
  White_gm_phi : RandomNumber  Variance=White_gm_phi  Seed=seed_ahrs  SampleTime=Ts_ahrs
  White_gm_psi : RandomNumber  Variance=White_gm_psi  Seed=seed_ahrs  SampleTime=Ts_ahrs
  White_gm_theta : RandomNumber  Variance=White_gm_theta  Seed=seed_ahrs  SampleTime=Ts_ahrs
  White_p : RandomNumber  Mean=mean_p  Variance=White_p  Seed=seed_ahrs  SampleTime=Ts_ahrs
  White_q : RandomNumber  Mean=mean_q  Variance=White_p  Seed=seed_ahrs  SampleTime=Ts_ahrs
  White_r : RandomNumber  Mean=mean_r  Variance=White_r  Seed=seed_ahrs  SampleTime=Ts_ahrs
  Zero-Order Hold{,1..8} (9 alike) : ZeroOrderHold  SampleTime=Ts_ahrs
  phi_out : Outport  VectorParamsAs1DForOutWhenUnconnected=off
  theta_out : Outport  Port=2  VectorParamsAs1DForOutWhenUnconnected=off
  psi_out : Outport  Port=3  VectorParamsAs1DForOutWhenUnconnected=off
  ax_out : Outport  Port=4  VectorParamsAs1DForOutWhenUnconnected=off
  ay_out : Outport  Port=5  VectorParamsAs1DForOutWhenUnconnected=off
  az_out : Outport  Port=6  VectorParamsAs1DForOutWhenUnconnected=off
  p_out : Outport  Port=7  VectorParamsAs1DForOutWhenUnconnected=off
  q_out : Outport  Port=8  VectorParamsAs1DForOutWhenUnconnected=off
  r_out : Outport  Port=9  VectorParamsAs1DForOutWhenUnconnected=off
  wires:
  Sum8/1 -> Integrator2/1
  Sum7/1 -> Integrator1/1
  q/1 -> Delay_ahrs7/1
  Gain2/1 -> Sum8/2
  White_p/1 -> Sum3/2
  p/1 -> Delay_ahrs6/1
  Integrator2/1 -> Gain2/1, Sum9/2
  Gain1/1 -> Sum7/2
  Gain/1 -> Sum6/2
  White_ax/1 -> Sum/2
  Integrator/1 -> Sum11/2, Gain/1
  Sum6/1 -> Integrator/1
  White_q/1 -> Sum4/2
  White_az/1 -> Sum2/2
  Integrator1/1 -> Sum10/2, Gain1/1
  Sum2/1 -> Zero-Order Hold5/1
  r/1 -> Delay_ahrs8/1
  White_r/1 -> Sum5/2
  White_ay/1 -> Sum1/2
  Sum5/1 -> Zero-Order Hold8/1
  ay/1 -> Delay_ahrs5/1
  Sum/1 -> Zero-Order Hold3/1
  phi/1 -> Delay_ahrs1/1
  psi/1 -> Delay_ahrs3/1
  Sum4/1 -> Zero-Order Hold7/1
  az/1 -> Delay_ahrs4/1
  ax/1 -> Delay_ahrs/1
  theta/1 -> Delay_ahrs2/1
  Sum3/1 -> Zero-Order Hold6/1
  Sum1/1 -> Zero-Order Hold4/1
  White_gm_phi/1 -> Sum8/1
  White_gm_theta/1 -> Sum7/1
  White_gm_psi/1 -> Sum6/1
  Sum9/1 -> Zero-Order Hold/1
  Sum10/1 -> Zero-Order Hold1/1
  Sum11/1 -> Zero-Order Hold2/1
  Delay_ahrs1/1 -> Sum9/1
  Delay_ahrs2/1 -> Sum10/1
  Delay_ahrs3/1 -> Sum11/1
  Delay_ahrs4/1 -> Sum2/1
  Delay_ahrs5/1 -> Sum1/1
  Delay_ahrs/1 -> Sum/1
  Delay_ahrs6/1 -> Sum3/1
  Delay_ahrs7/1 -> Sum4/1
  Delay_ahrs8/1 -> Sum5/1
  Zero-Order Hold/1 -> phi_out/1
  Zero-Order Hold1/1 -> theta_out/1
  Zero-Order Hold2/1 -> psi_out/1
  Zero-Order Hold3/1 -> ax_out/1
  Zero-Order Hold4/1 -> ay_out/1
  Zero-Order Hold5/1 -> az_out/1
  Zero-Order Hold6/1 -> p_out/1
  Zero-Order Hold7/1 -> q_out/1
  Zero-Order Hold8/1 -> r_out/1

== system v2021_10_27_Modello_SITL_AENEA_2020b/ 1/BMP 280 ==
  quota : Inport
  T0_ref : Inport  Port=2
  P_ref : Inport  Port=3
  Delay_bmp : TransportDelay  DelayTime=delay_bmp  InitialOutput=rho  TransDelayFeedthrough=on
  MATLAB Function1 : MATLAB Function  TreatAsAtomicUnit=on
  MATLAB Function3 : MATLAB Function  TreatAsAtomicUnit=on
  Sum : Sum  Inputs=|++
  White_press : RandomNumber  Variance=White_pressione  Seed=seed_baro  SampleTime=Ts_bmp
  Zero-Order Hold : ZeroOrderHold  SampleTime=Ts_bmp
  quota_out : Outport  VectorParamsAs1DForOutWhenUnconnected=off
  wires:
  quota/1 -> Delay_bmp/1
  P_ref/1 -> MATLAB Function3/3(P_ref), MATLAB Function1/3(P_ref)
  White_press/1 -> Sum/2
  MATLAB Function3/1(h_) -> Zero-Order Hold/1
  T0_ref/1 -> MATLAB Function3/2(T0ref), MATLAB Function1/2(T0ref)
  MATLAB Function1/1(P_) -> Sum/1
  Sum/1 -> MATLAB Function3/1(P)
  Delay_bmp/1 -> MATLAB Function1/1(h)
  Zero-Order Hold/1 -> quota_out/1

== system v2021_10_27_Modello_SITL_AENEA_2020b/ 1/GPS1 ==
  Lat : Inport
  Long : Inport  Port=2
  vel : Inport  Port=3
  head : Inport  Port=4
  Subsystem : Subsystem
  Subsystem1 : Subsystem
  Subsystem2 : Subsystem
  To Workspace : ToWorkspace  Commented=on  VariableName=Lat_out_cont  SaveFormat=Timeseries  SampleTime=-1
  To Workspace1 : ToWorkspace  Commented=on  VariableName=Long_out_cont  SaveFormat=Timeseries  SampleTime=-1
  Zero-Order Hold{,1..3} (4 alike) : ZeroOrderHold  SampleTime=Ts_gps
  Lat_out : Outport  VectorParamsAs1DForOutWhenUnconnected=off
  "Long_out " : Outport  Port=2  VectorParamsAs1DForOutWhenUnconnected=off
  V_n : Outport  Port=3  VectorParamsAs1DForOutWhenUnconnected=off
  V_e : Outport  Port=4  VectorParamsAs1DForOutWhenUnconnected=off
  wires:
  Long/1 -> Subsystem1/1(Long)
  Lat/1 -> Subsystem/1(Lat)
  head/1 -> Subsystem2/2(heading)
  vel/1 -> Subsystem2/1(Velocità)
  Zero-Order Hold3/1 -> V_e/1
  Zero-Order Hold2/1 -> V_n/1
  Zero-Order Hold1/1 -> "Long_out "/1
  Zero-Order Hold/1 -> Lat_out/1
  Subsystem2/2(V_e) -> Zero-Order Hold3/1
  Subsystem2/1("V_n ") -> Zero-Order Hold2/1
  Subsystem1/1(long_out) -> Zero-Order Hold1/1, To Workspace1/1
  Subsystem/1(Out1) -> Zero-Order Hold/1, To Workspace/1

== system v2021_10_27_Modello_SITL_AENEA_2020b/ 1/Sensore di pressione differenziale ==
  In1 : Inport
  Constant : Constant  Value=2
  Constant1 : Constant  Value=rho
  Divide : Product  Inputs=*/
  Product : Product
  Rate Transition23 : RateTransition  OutPortSampleTime=0.02
  Sqrt : Sqrt
  Sum3 : Sum  Inputs=++|
  White Noise1 : RandomNumber  DisableCoverage=on  Variance=3.9744  Seed=[23341]  SampleTime=sensori_RumoreSampleTime
  Zero-Order Hold19 : ZeroOrderHold  SampleTime=sensori_FreqCampionamento_pitot
  Out1 : Outport
  wires:
  White Noise1/1 -> Sum3/1
  Zero-Order Hold19/1 -> Rate Transition23/1  "deltaP"
  In1/1 -> Sum3/2
  Sum3/1 -> Zero-Order Hold19/1  "deltaP"
  Rate Transition23/1 -> Product/2  "deltaP"
  Constant/1 -> Product/1
  Product/1 -> Divide/1
  Constant1/1 -> Divide/2
  Divide/1 -> Sqrt/1
  Sqrt/1 -> Out1/1  "Ias"

== system v2021_10_27_Modello_SITL_AENEA_2020b/ 1/int1 ==
  In1 : Inport
  "INT16 " : Subsystem
  Out1 : Outport  VectorParamsAs1DForOutWhenUnconnected=off
  wires:
  In1/1 -> "INT16 "/1(<u>)
  "INT16 "/1(Out1) -> Out1/1

== system v2021_10_27_Modello_SITL_AENEA_2020b/ 1/int16 ==
  In1 : Inport
  "INT16 " : Subsystem
  Out1 : Outport  VectorParamsAs1DForOutWhenUnconnected=off
  wires:
  "INT16 "/1(Out1) -> Out1/1
  In1/1 -> "INT16 "/1(<u>)

== system v2021_10_27_Modello_SITL_AENEA_2020b/ 1/int16_rad  ==
  In1 : Inport
  Degrees to Radians : simulink_extras/Transformations/Degrees to Radians
  "INT16 " : Subsystem
  Radians to Degrees : simulink_extras/Transformations/Radians to Degrees
  Out1 : Outport  VectorParamsAs1DForOutWhenUnconnected=off
  wires:
  In1/1 -> Radians to Degrees/1
  "INT16 "/1(Out1) -> Degrees to Radians/1
  Degrees to Radians/1 -> Out1/1
  Radians to Degrees/1 -> "INT16 "/1(<u>)

== system v2021_10_27_Modello_SITL_AENEA_2020b/ 1/int16_rad 1 ==
  In1 : Inport
  Degrees to Radians : simulink_extras/Transformations/Degrees to Radians
  "INT16 " : Subsystem
  Radians to Degrees : simulink_extras/Transformations/Radians to Degrees
  Out1 : Outport  VectorParamsAs1DForOutWhenUnconnected=off
  wires:
  Degrees to Radians/1 -> Out1/1
  In1/1 -> Radians to Degrees/1
  Radians to Degrees/1 -> "INT16 "/1(<u>)
  "INT16 "/1(Out1) -> Degrees to Radians/1

== system v2021_10_27_Modello_SITL_AENEA_2020b/ 1/int16_rad 2 ==
  In1 : Inport
  Degrees to Radians : simulink_extras/Transformations/Degrees to Radians
  "INT16 " : Subsystem
  Radians to Degrees : simulink_extras/Transformations/Radians to Degrees
  Out1 : Outport  VectorParamsAs1DForOutWhenUnconnected=off
  wires:
  In1/1 -> Radians to Degrees/1
  "INT16 "/1(Out1) -> Degrees to Radians/1
  Radians to Degrees/1 -> "INT16 "/1(<u>)
  Degrees to Radians/1 -> Out1/1

== system v2021_10_27_Modello_SITL_AENEA_2020b/ 1/int16_rad 3 ==
  In1 : Inport
  Degrees to Radians : simulink_extras/Transformations/Degrees to Radians
  "INT16 " : Subsystem
  Radians to Degrees : simulink_extras/Transformations/Radians to Degrees
  Out1 : Outport  VectorParamsAs1DForOutWhenUnconnected=off
  wires:
  "INT16 "/1(Out1) -> Degrees to Radians/1
  In1/1 -> Radians to Degrees/1
  Radians to Degrees/1 -> "INT16 "/1(<u>)
  Degrees to Radians/1 -> Out1/1

== system v2021_10_27_Modello_SITL_AENEA_2020b/ 1/int16_rad 4 ==
  In1 : Inport
  Degrees to Radians : simulink_extras/Transformations/Degrees to Radians
  "INT16 " : Subsystem
  Radians to Degrees : simulink_extras/Transformations/Radians to Degrees
  Out1 : Outport  VectorParamsAs1DForOutWhenUnconnected=off
  wires:
  In1/1 -> Radians to Degrees/1
  "INT16 "/1(Out1) -> Degrees to Radians/1
  Radians to Degrees/1 -> "INT16 "/1(<u>)
  Degrees to Radians/1 -> Out1/1

== system v2021_10_27_Modello_SITL_AENEA_2020b/ 1/int16_rad 5 ==
  In1 : Inport
  Degrees to Radians : simulink_extras/Transformations/Degrees to Radians
  "INT16 " : Subsystem
  Radians to Degrees : simulink_extras/Transformations/Radians to Degrees
  Out1 : Outport  VectorParamsAs1DForOutWhenUnconnected=off
  wires:
  "INT16 "/1(Out1) -> Degrees to Radians/1
  In1/1 -> Radians to Degrees/1
  Radians to Degrees/1 -> "INT16 "/1(<u>)
  Degrees to Radians/1 -> Out1/1

== system v2021_10_27_Modello_SITL_AENEA_2020b/ 1/int2 ==
  In1 : Inport
  "INT16 " : Subsystem
  Out1 : Outport  VectorParamsAs1DForOutWhenUnconnected=off
  wires:
  "INT16 "/1(Out1) -> Out1/1
  In1/1 -> "INT16 "/1(<u>)

== system v2021_10_27_Modello_SITL_AENEA_2020b/ 1/single 1 ==
  <u> : Inport
  Data Type Conversion1 : DataTypeConversion  OutDataTypeStr=double  SaturateOnIntegerOverflow=off  RndMeth=Floor  LockScale=on
  Data Type Conversion2 : DataTypeConversion  OutDataTypeStr=single  SaturateOnIntegerOverflow=off  RndMeth=Floor  LockScale=on
  Degrees to Radians : simulink_extras/Transformations/Degrees to Radians
  Radians to Degrees : simulink_extras/Transformations/Radians to Degrees
  Out1 : Outport  VectorParamsAs1DForOutWhenUnconnected=off
  wires:
  Data Type Conversion1/1 -> Degrees to Radians/1
  <u>/1 -> Radians to Degrees/1
  Data Type Conversion2/1 -> Data Type Conversion1/1
  Radians to Degrees/1 -> Data Type Conversion2/1
  Degrees to Radians/1 -> Out1/1

== system v2021_10_27_Modello_SITL_AENEA_2020b/ 1/single 3 ==
  <u> : Inport
  Data Type Conversion1 : DataTypeConversion  OutDataTypeStr=double  SaturateOnIntegerOverflow=off  RndMeth=Floor  LockScale=on
  Data Type Conversion2 : DataTypeConversion  OutDataTypeStr=single  SaturateOnIntegerOverflow=off  RndMeth=Floor  LockScale=on
  Out1 : Outport  VectorParamsAs1DForOutWhenUnconnected=off
  wires:
  Data Type Conversion1/1 -> Out1/1
  <u>/1 -> Data Type Conversion2/1
  Data Type Conversion2/1 -> Data Type Conversion1/1

== system v2021_10_27_Modello_SITL_AENEA_2020b/ 1/single 4 ==
  <u> : Inport
  Data Type Conversion1 : DataTypeConversion  OutDataTypeStr=double  SaturateOnIntegerOverflow=off  RndMeth=Floor  LockScale=on
  Data Type Conversion2 : DataTypeConversion  OutDataTypeStr=single  SaturateOnIntegerOverflow=off  RndMeth=Floor  LockScale=on
  Degrees to Radians : simulink_extras/Transformations/Degrees to Radians
  Radians to Degrees : simulink_extras/Transformations/Radians to Degrees
  Out1 : Outport  VectorParamsAs1DForOutWhenUnconnected=off
  wires:
  Data Type Conversion2/1 -> Data Type Conversion1/1
  <u>/1 -> Radians to Degrees/1
  Data Type Conversion1/1 -> Degrees to Radians/1
  Radians to Degrees/1 -> Data Type Conversion2/1
  Degrees to Radians/1 -> Out1/1

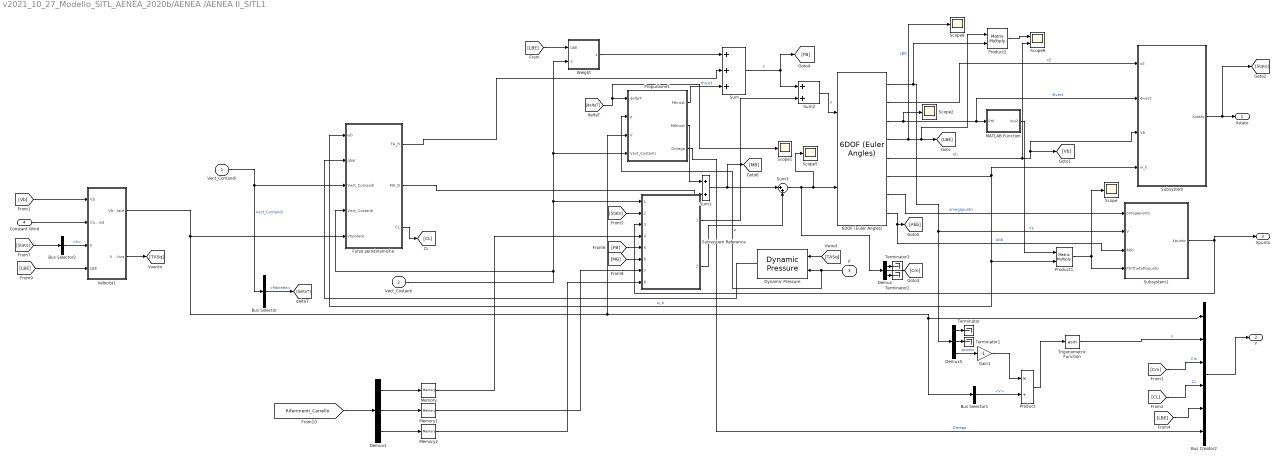
== system v2021_10_27_Modello_SITL_AENEA_2020b/AENEA /AENEA II_SITL1 ==
  Vect_Comandi : Inport
  Vect_Costanti : Inport  Port=2
  ρ : Inport  Port=3
  Constant Wind : Inport  Port=4
  6DOF (Euler Angles) : shared6dof/6DOF (Euler Angles)  units=Metric (MKS)  mtype=Fixed  rep=Euler Angles  xme_0=State0.Pos0  Vm_0=State0.Vb0  eul_0=State0.PHI0  pm_0=State0.Omega0  mass_0=m  mass_e=0.5  mass_f=2.0  inertia=I  inertia_e=eye(3)  inertia_f=2*eye(3)  k_quat=1.0  vre_flag=on  abi_flag=off  aMode=aMode  xme_statename=''  Vm_statename=''  eul_statename=''  quat_statename=''  pm_statename=''  mass_statename=''
      settings: SourceProductBaseCode=AE,PW,DR,MT,VE
  Bus Creator2 : BusCreator  Inputs=6
  Bus Selector : BusSelector  OutputSignals=Manetta
  Bus Selector1 : BusSelector  OutputSignals=V
  Bus Selector2 : BusSelector  OutputSignals=xyz.h
  Demux : Demux  Outputs=3
  Demux1 : Demux  Outputs=3
  Demux5 : Demux  Outputs=3
  Dynamic Pressure : aerolibasang/Dynamic Pressure
  Forze aerodinamiche : Subsystem
  Gain1 : Gain  Gain=-1
  MATLAB Function : MATLAB Function  TreatAsAtomicUnit=on
  Memory : Memory
  Memory1 : Memory
  Memory2 : Memory
  Product : Product  Inputs=*/
  Product1 : Product  Multiplication=Matrix(*)
  Product2 : Product  Multiplication=Matrix(*)  InputSameDT=on  RndMeth=Zero  SaturateOnIntegerOverflow=on  OutDataTypeStr=Inherit: Same as first input
  Propulsione1 : Subsystem
  Scope{,1..2,5,8} (5 alike) : Scope
  Scope9 : Scope  NumInputPorts=2
  Subsystem : Subsystem
  Subsystem Reference : Subsystem  ReferencedSubsystem=v2021_10_27_Gear
  Subsystem1 : Subsystem
  Sum : Sum  Inputs=+++
  Sum1 : Sum
  Sum2 : Sum
  Sum3 : Sum  Inputs=|++
  Terminator{,1..3} (4 alike) : Terminator
  Trigonometric Function : Trigonometry  Operator=asin
  Velocità1 : Subsystem
  Weight : Subsystem
  Xstato : Outport  VectorParamsAs1DForOutWhenUnconnected=off
  Y : Outport  Port=2  VectorParamsAs1DForOutWhenUnconnected=off
  Xpunto : Outport  Port=3  VectorParamsAs1DForOutWhenUnconnected=off
  wires:
  Sum/1 -> Sum2/1, [FB]  "F"
  6DOF (Euler Angles)/5 -> Scope9/2, Subsystem/3(Vb), [Vb]  "Vb"
  6DOF (Euler Angles)/6 -> Forze aerodinamiche/1(ωb), Product1/2, Subsystem/4(ω_b)  "ω_b"
  6DOF (Euler Angles)/4 -> Scope8/1, Product2/1, [LBE]  "LBE"
  Forze aerodinamiche/1(FA_B) -> Sum/2
  Forze aerodinamiche/2(MA_B) -> Sum1/2
  6DOF (Euler Angles)/1 -> Product2/2, Demux5/1, Subsystem1/2(V)  "Ve"
  Dynamic Pressure/1 -> Forze aerodinamiche/2(qbar)
  Sum1/1 -> Sum3/1, [MB]
  Weight/1("Forzapeso ") -> Sum/1
  [LBE] -> Weight/1(LBE)
  Vect_Comandi/1 -> Bus Selector/1, Forze aerodinamiche/3(Vect_Comandi)  "Vect_Comandi"
  Bus Selector/1 -> [deltaT]  "<Manetta>"
  Bus Creator2/1 -> Y/1
  Gain1/1 -> Product/1
  Product/1 -> Trigonometric Function/1
  Trigonometric Function/1 -> Bus Creator2/2  "γ"
  ρ/1 -> Propulsione1/2(ρ), Dynamic Pressure/2  "ρ"
  Velocità1/1(Vbpolare) -> Propulsione1/3(V), Bus Selector1/1, Bus Creator2/1, Forze aerodinamiche/5("Vbpolare ")
  [Vb] -> Velocità1/1(Vb)
  6DOF (Euler Angles)/3 -> Scope2/1, Subsystem/2(Φvect), MATLAB Function/1(PHI)  "Φvect"
  Bus Selector1/1 -> Product/2  "<V>"
  Constant Wind/1 -> Velocità1/2(Constant Wind)
  Forze aerodinamiche/3(CL) -> [CL]
  [Cm] -> Bus Creator2/3  "Cm"
  [CL] -> Bus Creator2/4  "CL"
  6DOF (Euler Angles)/2 -> Subsystem/1(xE)  "xE"
  Subsystem/1("Xstato ") -> [Stato], Xstato/1
  Demux5/2 -> Terminator1/1
  Demux5/1 -> Terminator/1
  Demux5/3 -> Gain1/1  "zpunto"
  6DOF (Euler Angles)/7 -> Subsystem1/1(omegapunto)  "omegapunto"
  6DOF (Euler Angles)/8 -> [Abb], Subsystem1/3(Abb)  "Abb"
  Subsystem1/1(Xpunto) -> Xpunto/1, Subsystem Reference/3
  Product1/1 -> Subsystem1/4("PhiThetaPsipunto "), Scope/1
  MATLAB Function/1(invR) -> Product1/1
  [deltaT] -> Propulsione1/1("deltaT "), Scope1/1
  Vect_Costanti/1 -> Forze aerodinamiche/4(Vect_Costanti), Subsystem Reference/1, Weight/2(Vect_Costanti), Propulsione1/4(Vect_Costanti)
  Propulsione1/2(Mthrust) -> Sum1/1
  Propulsione1/1("Fthrust ") -> Sum/3  "thrust"
  Demux/2 -> [Cm]
  Demux/3 -> Terminator2/1
  Demux/1 -> Terminator3/1
  [LBE] -> Bus Creator2/5
  Propulsione1/3(Omega) -> Bus Creator2/6  "Omega"
  Velocità1/2("V effettiva ") -> [TASq]
  [TASq] -> Dynamic Pressure/1
  Sum2/1 -> 6DOF (Euler Angles)/1  "F"
  [FB] -> Subsystem Reference/5
  Subsystem Reference/1 -> Sum2/2
  Subsystem Reference/2 -> Sum3/2
  Sum3/1 -> Demux/1, Scope5/1, 6DOF (Euler Angles)/2
  [MB] -> Subsystem Reference/6
  [Stato] -> Subsystem Reference/2
  [Stato] -> Bus Selector2/1
  Bus Selector2/1 -> Velocità1/3(h)  "<h>"
  [LBE] -> Velocità1/4(LBE)
  Product2/1 -> Scope9/1
  Demux1/3 -> Memory2/1
  Memory2/1 -> Subsystem Reference/8
  [Riferimenti_Carrello] -> Demux1/1
  Demux1/1 -> Memory/1
  Demux1/2 -> Memory1/1
  Memory/1 -> Subsystem Reference/4
  Memory1/1 -> Subsystem Reference/7
